simulink model "Trigger_Every_5ms_Edited"  (R2018a)
settings: Solver=FixedStepDiscrete  StartTime=0.0  StopTime=10.0  RelTol=1e-3
settings Model: Creator=Moataz  LastModifiedBy=Moataz
settings OptimizationCC: DefaultParameterBehavior=Inlined  EnhancedBackFolding=on  PassReuseOutputArgsAs=Individual arguments  OptimizeBlockOrder=speed  DifferentSizesBufferReuse=on  OptimizationCustomize=off
settings DebuggingCC: ParameterTunabilityLossMsg=error
settings SFSimCC: MATLABDynamicMemAlloc=off
settings SFSimCC: SimCustomHeaderCode=|
  | #include	"STD_TYPES.h"
  | #include	"BIT_MATH.h"
  | #include	"Dio_interface.h"
  | #include	"Dio_private.h"
  | #include  "LED.h"
  | #include  "Switch.h"
settings SFSimCC: SimUserSources=|
  | Dio_program.c
  | LED.c
  | Switch.c
settings RTWCC: SystemTargetFile=ert.tlc  GenCodeOnly=on  TemplateMakefile=ert_default_tmf  GenerateReport=on  RTWUseSimCustomCode=on  IncludeHyperlinkInReport=on  LaunchReport=on  GenerateTraceInfo=on  GenerateTraceReport=on  GenerateTraceReportSl=on  GenerateTraceReportSf=on  GenerateTraceReportEml=on
settings RTWCC: CustomHeaderCode=|
  | #include	"STD_TYPES.h"
  | #include	"BIT_MATH.h"
  | #include	"Dio_interface.h"
  | #include	"Dio_private.h"
  | #include  "LED.h"
  | #include  "Switch.h"
settings RTWCC: CustomSource=|
  | Dio_program.c
  | LED.c
  | Switch.c
settings CodeAppCC: ForceParamTrailComments=on  IgnoreCustomStorageClasses=off  OperatorAnnotations=on  SimulinkDataObjDesc=on  SFDataObjDesc=on  InsertBlockDesc=on
settings ERTTargetCC: TargetLangStandard=C99 (ISO)  GenerateSampleERTMain=on  InlinedParameterPlacement=NonHierarchical  ERTCustomFileTemplate=example_file_process.tlc

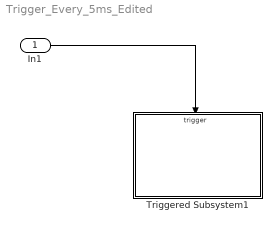
== system Trigger_Every_5ms_Edited ==
  In1 : Inport  OutputFunctionCall=on
  Triggered Subsystem1 : Subsystem  TreatAsAtomicUnit=on
  wires:
  In1/1 -> Triggered Subsystem1/Trigger

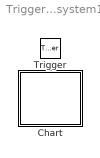
== system Trigger_Every_5ms_Edited/Triggered Subsystem1 ==
  Trigger : TriggerPort  TriggerType=function-call  VariantControl=Variant
  Chart : Stateflow chart  TreatAsAtomicUnit=on

== stateflow chart Trigger_Every_5ms_Edited/Triggered Subsystem1/Chart ==
  (default) -> (junction 115) : /* SwitchState */
      | {Read_Switch = ReadSwitch(SWITCH_1);}
  (junction 115) -> (junction 116) [order 1] : [Read_Switch==1]
  (junction 115) -> (junction 118) [order 2] : {Switch_Pressed=0;}
  (junction 116) -> (junction 113) : {Switch_Pressed=1;}
  (junction 113) -> (junction 118)
  (junction 118) -> (junction 130) : /* LEDState */
  (junction 130) -> (junction 129) [order 1] : [Switch_Pressed==1]
  (junction 130) -> (junction 128) [order 2] : {Led_TurnOff(LED_1);}
  (junction 129) -> (junction 127) : {Led_TurnOn(LED_1);}
  (junction 127) -> (junction 128)
  (junction 128) -> (junction 131)
  data: Read_Switch local boolean; Switch_Pressed local boolean
